simulink library "lib_converters"  (R2020b)
settings: Solver=VariableStepAuto  StartTime=0.0  StopTime=10.0  RelTol=1e-3
undefined symbols (not defined in the file): C_sc, DiscIntNeverNeededParam
libraries: powerlib x170, simulink x12, $bdroot x6, powerlib_meascontrol x3
(part 3 of 3)

== system lib_converters/Boost - FC/Discrete PI Controller3 ==
  note: Pierre Giroux, Gilbert Sybille
      | Power System Simulation Laboratory
      | IREQ, Hydro-Quebc
  note: Discrete PID Controller
  Error : Inport  SampleTime=Ts
  Discrete-Time Integrator : DiscreteIntegrator  InitialCondition=Init  SampleTime=Ts  LimitOutput=on  UpperSaturationLimit=UpperLimit  LowerSaturationLimit=LowerLimit  ICPrevOutput=DiscIntNeverNeededParam  ICPrevScaledInput=DiscIntNeverNeededParam
  Kp4 : Gain  Gain=Kp  SaturateOnIntegerOverflow=on  SampleTime=Ts  OutDataTypeStr=Inherit: Same as input  ParamDataTypeStr=Inherit: Same as input
  Kp5 : Gain  Gain=Ki  SaturateOnIntegerOverflow=on  SampleTime=Ts  OutDataTypeStr=Inherit: Same as input  ParamDataTypeStr=Inherit: Same as input
  Saturation2 : Saturate  UpperLimit=UpperLimit  LowerLimit=LowerLimit  SampleTime=Ts
  Sum6 : Sum  InputSameDT=on  SaturateOnIntegerOverflow=on  SampleTime=Ts  OutDataTypeStr=Inherit: Same as first input
  Zero-Order Hold : ZeroOrderHold  SampleTime=Ts
  Out : Outport  SampleTime=Ts  InitialOutput=0  VectorParamsAs1DForOutWhenUnconnected=off
  wires:
  Error/1 -> Kp4/1, Kp5/1
  Sum6/1 -> Saturation2/1
  Kp5/1 -> Discrete-Time Integrator/1
  Kp4/1 -> Zero-Order Hold/1
  Discrete-Time Integrator/1 -> Sum6/2
  Saturation2/1 -> Out/1
  Zero-Order Hold/1 -> Sum6/1

== system lib_converters/Boost - FC/Discrete PI Controller4 ==
  note: Discrete PID Controller
  note: Pierre Giroux, Gilbert Sybille
      | Power System Simulation Laboratory
      | IREQ, Hydro-Quebc
  Error : Inport  SampleTime=Ts
  Discrete-Time Integrator : DiscreteIntegrator  InitialCondition=Init  SampleTime=Ts  LimitOutput=on  UpperSaturationLimit=UpperLimit  LowerSaturationLimit=LowerLimit  ICPrevOutput=DiscIntNeverNeededParam  ICPrevScaledInput=DiscIntNeverNeededParam
  Kp4 : Gain  Gain=Kp  SaturateOnIntegerOverflow=on  SampleTime=Ts  OutDataTypeStr=Inherit: Same as input  ParamDataTypeStr=Inherit: Same as input
  Kp5 : Gain  Gain=Ki  SaturateOnIntegerOverflow=on  SampleTime=Ts  OutDataTypeStr=Inherit: Same as input  ParamDataTypeStr=Inherit: Same as input
  Saturation2 : Saturate  UpperLimit=UpperLimit  LowerLimit=LowerLimit  SampleTime=Ts
  Sum6 : Sum  InputSameDT=on  SaturateOnIntegerOverflow=on  SampleTime=Ts  OutDataTypeStr=Inherit: Same as first input
  Zero-Order Hold : ZeroOrderHold  SampleTime=Ts
  Out : Outport  SampleTime=Ts  InitialOutput=0  VectorParamsAs1DForOutWhenUnconnected=off
  wires:
  Zero-Order Hold/1 -> Sum6/1
  Saturation2/1 -> Out/1
  Discrete-Time Integrator/1 -> Sum6/2
  Kp4/1 -> Zero-Order Hold/1
  Kp5/1 -> Discrete-Time Integrator/1
  Sum6/1 -> Saturation2/1
  Error/1 -> Kp5/1, Kp4/1

== system lib_converters/Boost - PV/Control ==
  Vcom : Inport
  Icom : Inport  Port=2
  Vout : Inport  Port=3
  Iout : Inport  Port=4
  Vpv_in : Inport  Port=5
  IL : Inport  Port=6
  g : Inport  Port=7
  IR : Inport  Port=8
  Cascade-control : Subsystem  VariantControl=Cascade-control
  MPPT : Subsystem  VariantControl=MPPT
  Duty Cycle PV conv : Outport

== system lib_converters/Boost - PV - chsvar/Subsystem1 ==
  Vcom : Inport
  Icom : Inport  Port=2
  Vout : Inport  Port=3
  Iout : Inport  Port=4
  Vpv_in : Inport  Port=5
  IL : Inport  Port=6
  g : Inport  Port=7
  IR : Inport  Port=8
  Control : Inport  Port=9
  MATLAB Function : MATLAB Function  TreatAsAtomicUnit=on
  Saturation : Saturate  UpperLimit=1
  Subsystem : Subsystem
  Subsystem1 : Subsystem
  DutyCycle : Outport
  wires:
  Subsystem/1(Duty Cycle PV conv) -> MATLAB Function/2(mppt)
  Subsystem1/1(Duty Cycle PV conv) -> MATLAB Function/3(cascade)
  IR/1 -> [IR]
  g/1 -> [g]
  IL/1 -> [IL]
  Vpv_in/1 -> [Vpv_in]
  Iout/1 -> [Iout]
  Vout/1 -> [Vout]
  Icom/1 -> [Icom]
  Vcom/1 -> [Vcom]
  [Vcom] -> Subsystem/1(Vcom)
  [IR] -> Subsystem/8(IR)
  [Vout] -> Subsystem/3(Vout)
  [Icom] -> Subsystem/2(Icom)
  [g] -> Subsystem/7(g)
  [IL] -> Subsystem/6(IL)
  [Vpv_in] -> Subsystem/5(Vpv_in)
  [Iout] -> Subsystem/4(Iout)
  [Iout] -> Subsystem1/4(Iout)
  [Vpv_in] -> Subsystem1/5(Vpv_in)
  [IL] -> Subsystem1/6(IL)
  [g] -> Subsystem1/7(g)
  [Icom] -> Subsystem1/2(Icom)
  [Vout] -> Subsystem1/3(Vout)
  [IR] -> Subsystem1/8(IR)
  [Vcom] -> Subsystem1/1(Vcom)
  Saturation/1 -> DutyCycle/1
  MATLAB Function/1(d) -> Saturation/1
  Control/1 -> MATLAB Function/1(u1)

== system lib_converters/Boost FC avg-swh/Converter type ==
  g : Inport
  D : Inport  Port=2
  n : Inport  Port=3
  Avg : Subsystem  VariantControl=Choice
  Swh : Subsystem  VariantControl=Choice_1
  L+ : PMIOPort  Side=Left
  L- : PMIOPort  Port=2  Side=Left
  H+ : PMIOPort  Port=3  Side=Right
  H- : PMIOPort  Port=4  Side=Right
  VL : Outport
  IL : Outport  Port=2
  IR : Outport  Port=3
  VH : Outport  Port=4

== system lib_converters/Boost FC swh/Converter type ==
  g : Inport
  D : Inport  Port=2
  n : Inport  Port=3
  Avg : Subsystem  VariantControl=Choice
  Swh : Subsystem  VariantControl=Choice_1
  L+ : PMIOPort  Side=Left
  L- : PMIOPort  Port=2  Side=Left
  H+ : PMIOPort  Port=3  Side=Right
  H- : PMIOPort  Port=4  Side=Right
  VL : Outport
  IL : Outport  Port=2
  IR : Outport  Port=3
  VH : Outport  Port=4

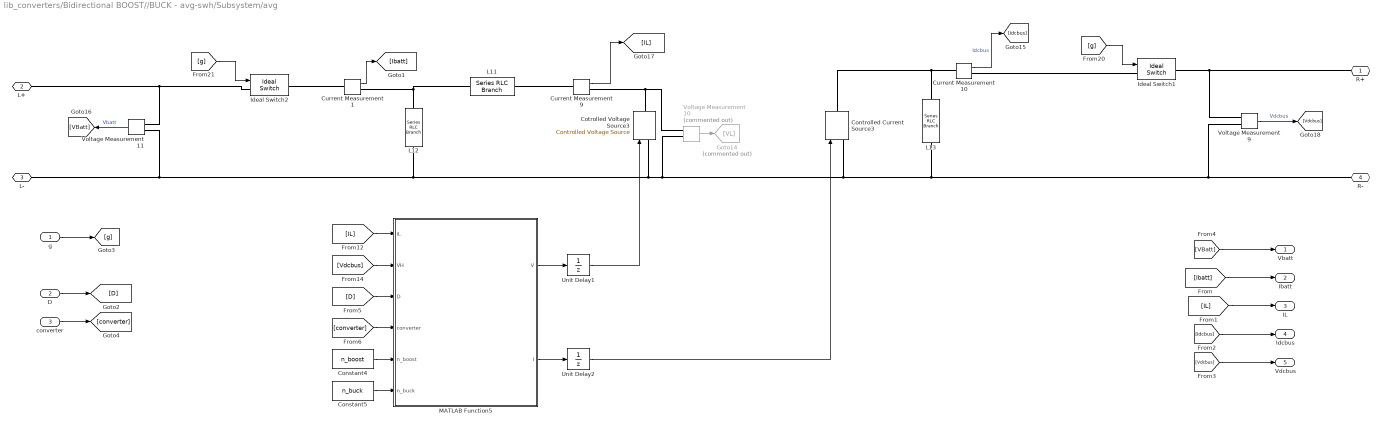
== system lib_converters/Bidirectional BOOST//BUCK - avg-swh/Subsystem/avg ==
  g : Inport
  D : Inport  Port=2
  converter : Inport  Port=3
  Constant4 : Constant  Value=n_boost
  Constant5 : Constant  Value=n_buck
  Controlled Current Source3 : powerlib/Electrical Sources/Controlled Current Source  Initialize=on  Source_Type=DC  Amplitude=0  Phase=0  Frequency=0  Measurements=None
  Cotrolled Voltage Source3 : powerlib/Electrical Sources/Controlled Voltage Source  Initialize=on  Source_Type=DC  Amplitude=0  Phase=0  Frequency=0  Measurements=None
  Current Measurement1 : powerlib/Measurements/Current Measurement  PhasorSimulation=off  OutputType=Complex  PSBequivalent=0
  Current Measurement10 : powerlib/Measurements/Current Measurement  PhasorSimulation=off  OutputType=Complex  PSBequivalent=0
  Current Measurement9 : powerlib/Measurements/Current Measurement  PhasorSimulation=off  OutputType=Complex  PSBequivalent=0
  Goto14 : Goto  Commented=on  GotoTag=VL
  Ideal Switch1 : powerlib/Power Electronics/Ideal Switch  Ron=0.001  Lon=0  IC=0  Rs=1e5  Cs=inf  Measurements=off
  Ideal Switch2 : powerlib/Power Electronics/Ideal Switch  Ron=0.001  Lon=0  IC=0  Rs=1e5  Cs=inf  Measurements=off
  L11 : powerlib/Elements/Series RLC Branch  LConnTagsString=__new0  RConnTagsString=__new0  BranchType=L  Resistance=0.3  Inductance=L  SetiL0=off  InitialCurrent=100  Capacitance=100e-6  Setx0=off  InitialVoltage=0  Measurements=None
  L12 : powerlib/Elements/Series RLC Branch  LConnTagsString=__new0  RConnTagsString=__new0  BranchType=RC  Resistance=0.01  Inductance=100e-6  SetiL0=off  InitialCurrent=100  Capacitance=Co  Setx0=off  InitialVoltage=0  Measurements=None
  L13 : powerlib/Elements/Series RLC Branch  LConnTagsString=__new0  RConnTagsString=__new0  BranchType=RC  Resistance=0.01  Inductance=100e-6  SetiL0=off  InitialCurrent=100  Capacitance=Co  Setx0=off  InitialVoltage=0  Measurements=None
  MATLAB Function5 : MATLAB Function  TreatAsAtomicUnit=on
  Unit Delay1 : UnitDelay  SampleTime=Ts  HasFrameUpgradeWarning=on
  Unit Delay2 : UnitDelay  SampleTime=Ts  HasFrameUpgradeWarning=on
  Voltage Measurement10 : powerlib/Measurements/Voltage Measurement  Commented=on  PhasorSimulation=off  OutputType=Complex  PSBequivalent=0
  Voltage Measurement11 : powerlib/Measurements/Voltage Measurement  PhasorSimulation=off  OutputType=Complex  PSBequivalent=0
  Voltage Measurement9 : powerlib/Measurements/Voltage Measurement  PhasorSimulation=off  OutputType=Complex  PSBequivalent=0
  R+ : PMIOPort  Side=Right
  L+ : PMIOPort  Port=2  Side=Left
  L- : PMIOPort  Port=3  Side=Left
  R- : PMIOPort  Port=4  Side=Right
  Vbatt : Outport
  Ibatt : Outport  Port=2
  IL : Outport  Port=3
  Idcbus : Outport  Port=4
  Vdcbus : Outport  Port=5
  wires:
  [g] -> Ideal Switch1/1
  MATLAB Function5/2(I) -> Unit Delay2/1
  Current Measurement1/1 -> [Ibatt]
  [D] -> MATLAB Function5/3(D)
  Voltage Measurement11/1 -> [VBatt]  "Vbatt"
  Unit Delay2/1 -> Controlled Current Source3/1
  Voltage Measurement9/1 -> [Vdcbus]  "Vdcbus"
  [converter] -> MATLAB Function5/4(converter)
  [Vdcbus] -> MATLAB Function5/2(VH)
  Constant4/1 -> MATLAB Function5/5(n_boost)
  [g] -> Ideal Switch2/1
  [IL] -> MATLAB Function5/1(iL)
  MATLAB Function5/1(V) -> Unit Delay1/1
  Unit Delay1/1 -> Cotrolled Voltage Source3/1
  Current Measurement9/1 -> [IL]
  Voltage Measurement10/1 -> Goto14/1
  Constant5/1 -> MATLAB Function5/6(n_buck)
  Current Measurement10/1 -> [Idcbus]  "Idcbus"
  g/1 -> [g]
  converter/1 -> [converter]
  D/1 -> [D]
  [VBatt] -> Vbatt/1
  [Ibatt] -> Ibatt/1
  [IL] -> IL/1
  [Idcbus] -> Idcbus/1
  [Vdcbus] -> Vdcbus/1
  connections:
  Voltage Measurement9/LConn2 -- R-/RConn1 -- L13/RConn1 -- Controlled Current Source3/LConn1 -- Voltage Measurement10/LConn2 -- Cotrolled Voltage Source3/LConn1 -- L-/RConn1 -- Voltage Measurement11/LConn2 -- L12/RConn1
  Controlled Current Source3/RConn1 -- Current Measurement10/LConn1 -- L13/LConn1
  Current Measurement1/RConn1 -- L12/LConn1 -- L11/RConn1
  Voltage Measurement10/LConn1 -- Cotrolled Voltage Source3/RConn1 -- Current Measurement9/RConn1
  R+/RConn1 -- Ideal Switch1/RConn1 -- Voltage Measurement9/LConn1
  Ideal Switch2/LConn1 -- L+/RConn1 -- Voltage Measurement11/LConn1
  Ideal Switch1/LConn1 -- Current Measurement10/RConn1
  Current Measurement9/LConn1 -- L11/LConn1
  Ideal Switch2/RConn1 -- Current Measurement1/LConn1

== system lib_converters/Bidirectional BOOST//BUCK - avg-swh/Subsystem/swh ==
  g : Inport
  D : Inport  Port=2
  converter : Inport  Port=3
  Current Measurement1 : powerlib/Measurements/Current Measurement  PhasorSimulation=off  OutputType=Complex  PSBequivalent=0
  Current Measurement10 : powerlib/Measurements/Current Measurement  PhasorSimulation=off  OutputType=Complex  PSBequivalent=0
  Current Measurement9 : powerlib/Measurements/Current Measurement  PhasorSimulation=off  OutputType=Complex  PSBequivalent=0
  Ideal Switch1 : powerlib/Power Electronics/Ideal Switch  Ron=0.001  Lon=0  IC=0  Rs=1e5  Cs=inf  Measurements=off
  Ideal Switch2 : powerlib/Power Electronics/Ideal Switch  Ron=0.001  Lon=0  IC=0  Rs=1e5  Cs=inf  Measurements=off
  L11 : powerlib/Elements/Series RLC Branch  LConnTagsString=__new0  RConnTagsString=__new0  BranchType=L  Resistance=0.3  Inductance=L  SetiL0=off  InitialCurrent=100  Capacitance=100e-6  Setx0=off  InitialVoltage=0  Measurements=None
  L12 : powerlib/Elements/Series RLC Branch  LConnTagsString=__new0  RConnTagsString=__new0  BranchType=RC  Resistance=0.01  Inductance=100e-6  SetiL0=off  InitialCurrent=100  Capacitance=Co  Setx0=off  InitialVoltage=0  Measurements=None
  L13 : powerlib/Elements/Series RLC Branch  LConnTagsString=__new0  RConnTagsString=__new0  BranchType=RC  Resistance=0.01  Inductance=100e-6  SetiL0=off  InitialCurrent=100  Capacitance=Co  Setx0=off  InitialVoltage=0  Measurements=None
  Mosfet : powerlib/Power Electronics/Mosfet  Ron=0.1  Lon=0  Rd=0.01  Vfd=0  IC=0  Rs=1e5  Cs=inf  Measurements=on
  Mosfet1 : powerlib/Power Electronics/Mosfet  Ron=0.1  Lon=0  Rd=0.01  Vfd=0  IC=0  Rs=1e5  Cs=inf  Measurements=on
  NOT : Logic  Operator=NOT  IconShape=distinctive  AllPortsSameDT=off  OutDataTypeStr=boolean
  PWM Generator (DC-DC) : powerlib_meascontrol/Pulse & Signal Generators/PWM Generator (DC-DC)  Fsw=100000  Ts=Ts
  Product : Product
  Product1 : Product
  Voltage Measurement11 : powerlib/Measurements/Voltage Measurement  PhasorSimulation=off  OutputType=Complex  PSBequivalent=0
  Voltage Measurement9 : powerlib/Measurements/Voltage Measurement  PhasorSimulation=off  OutputType=Complex  PSBequivalent=0
  R+ : PMIOPort  Side=Right
  L+ : PMIOPort  Port=2  Side=Left
  L- : PMIOPort  Port=3  Side=Left
  R- : PMIOPort  Port=4  Side=Right
  Vbatt : Outport
  Ibatt : Outport  Port=2
  IL : Outport  Port=3
  Idcbus : Outport  Port=4
  Vdcbus : Outport  Port=5
  wires:
  Current Measurement9/1 -> [IL]
  [g] -> Ideal Switch2/1
  Voltage Measurement11/1 -> [VBatt]  "Vbatt"
  [g] -> Ideal Switch1/1
  Voltage Measurement9/1 -> [Vdcbus]  "Vdcbus"
  Current Measurement1/1 -> [Ibatt]
  D/1 -> [D]
  Current Measurement10/1 -> [Idcbus]  "Idcbus"
  g/1 -> [g]
  [Idcbus] -> Idcbus/1
  [Ibatt] -> Ibatt/1
  [Vdcbus] -> Vdcbus/1
  [IL] -> IL/1
  [VBatt] -> Vbatt/1
  converter/1 -> [converter]
  [D] -> PWM Generator (DC-DC)/1
  PWM Generator (DC-DC)/1 -> Product1/1, Product/1
  [converter] -> NOT/1, Product/2
  NOT/1 -> Product1/2
  Product1/1 -> Mosfet1/1
  Product/1 -> Mosfet/1
  connections:
  L12/RConn1 -- Mosfet1/RConn1 -- L13/RConn1 -- R-/RConn1 -- Voltage Measurement9/LConn2 -- L-/RConn1 -- Voltage Measurement11/LConn2
  R+/RConn1 -- Ideal Switch1/RConn1 -- Voltage Measurement9/LConn1
  Current Measurement1/RConn1 -- L12/LConn1 -- L11/RConn1
  Ideal Switch2/LConn1 -- L+/RConn1 -- Voltage Measurement11/LConn1
  L13/LConn1 -- Current Measurement10/LConn1 -- Mosfet/LConn1
  Current Measurement9/LConn1 -- L11/LConn1
  Ideal Switch1/LConn1 -- Current Measurement10/RConn1
  Ideal Switch2/RConn1 -- Current Measurement1/LConn1
  Mosfet1/LConn1 -- Mosfet/RConn1 -- Current Measurement9/RConn1

== system lib_converters/Boost - PV/Control/Cascade-control ==
  note: Current Regulator
  note: Voltage Regulator
  Vcom : Inport
  Icom : Inport  Port=2
  Vout : Inport  Port=3
  Iout : Inport  Port=4
  Vpv_in : Inport  Port=5
  IL : Inport  Port=6
  g : Inport  Port=7
  IR : Inport  Port=8
  Constant : Constant
  Constant1 : Constant  Value=0
  Constant8 : Constant  Value=n
  Discrete PI Controller3 : Subsystem  DialogController=POWERSYS.PowerSysDialog  mask(Discrete PI Controller){Kp=Kpv, Ki=Kiv, Par_Limits=[0.5 -0.5], Init=0, Ts=Ts}
      mask prompts: Kp "Proportional gain (Kp):"; Ki "Integral gain (Ki):"; Par_Limits "Output limits: [ Upper   Lower ]"; Init "Output initial value:"; Ts "Sample time:"
      mask help: This block implements a discrete PI controller.
      mask init:
      | UpperLimit=Par_Limits(1);
      | LowerLimit=Par_Limits(2);
      | power_initmask();
      mask Help: This block is part of a subset of blocks in the Extras library that does not have documentation associated with it, other than the block mask description.
      mask Display: disp('PI');
  Discrete PI Controller4 : Subsystem  DialogController=POWERSYS.PowerSysDialog  mask(Discrete PI Controller){Kp=Kpi, Ki=Kii, Par_Limits=[50 -50], Init=0, Ts=Ts}
      mask prompts: Kp "Proportional gain (Kp):"; Ki "Integral gain (Ki):"; Par_Limits "Output limits: [ Upper   Lower ]"; Init "Output initial value:"; Ts "Sample time:"
      mask help: This block implements a discrete PI controller.
      mask init:
      | UpperLimit=Par_Limits(1);
      | LowerLimit=Par_Limits(2);
      | power_initmask();
      mask Help: This block is part of a subset of blocks in the Extras library that does not have documentation associated with it, other than the block mask description.
      mask Display: disp('PI');
  Divide : Product  Inputs=*/  SampleTime=Ts
  Divide1 : Product  Inputs=*/  SampleTime=Ts
  Product : Product  RndMeth=Zero
  Product1 : Product  RndMeth=Zero
  Product2 : Product  RndMeth=Zero
  Saturation : Saturate  UpperLimit=inf  LowerLimit=0.01  SampleTime=Ts
  Saturation Dynamic : simulink/Discontinuities/Saturation Dynamic  OutMin=[]  OutMax=[]  OutDataTypeStr=Inherit: Same as second input  OutDataType=fixdt(1, 16)  OutScaling=2^-10  DoSatur=off
  Saturation1 : Saturate  UpperLimit=1  LowerLimit=0  SampleTime=Ts
  Saturation2 : Saturate  UpperLimit=inf  LowerLimit=0.01  SampleTime=Ts
  Sum : Sum  Inputs=|+-
  Sum1 : Sum  Inputs=|-+
  Sum2 : Sum  Inputs=|-+
  Sum3 : Sum  Inputs=|+-
  Sum4 : Sum  Inputs=|++
  Duty Cycle PV conv : Outport
  wires:
  Vout/1 -> [VH]
  Iout/1 -> ?
  IL/1 -> [IL]
  Vpv_in/1 -> [VL]
  Saturation1/1 -> Duty Cycle PV conv/1  "Duty Cycle PV conv"
  Vcom/1 -> Sum3/1
  Constant8/1 -> Product2/2
  Divide/1 -> Sum2/1
  Icom/1 -> Product1/1
  Discrete PI Controller3/1(Out) -> Sum4/1
  Product2/1 -> Saturation2/1
  Sum4/1 -> Product/1
  [IL] -> Sum/2
  Saturation/1 -> Divide/2
  Saturation2/1 -> Divide1/2
  [VH] -> Saturation/1
  Saturation Dynamic/1 -> [ILref]
  [IR] -> Sum4/2
  Divide1/1 -> Product/2
  [VL] -> Sum1/2
  [ILref] -> Sum/1
  [VH] -> Divide1/1
  [VH] -> Sum3/2
  Product/1 -> Saturation Dynamic/2
  Sum/1 -> Discrete PI Controller4/1(Error)
  Discrete PI Controller4/1(Out) -> Sum1/1
  Constant1/1 -> Saturation Dynamic/3
  Sum2/1 -> Saturation1/1
  Constant/1 -> Sum2/2
  [g] -> Product1/2
  Sum3/1 -> Discrete PI Controller3/1(Error)
  Sum1/1 -> Divide/1
  Product1/1 -> Saturation Dynamic/1
  [VL] -> Product2/1
  IR/1 -> [IR]
  g/1 -> [g]

== system lib_converters/Boost - PV/Control/MPPT ==
  Vcom : Inport
  Icom : Inport  Port=2
  Vout : Inport  Port=3
  Iout : Inport  Port=4
  Vpv_in : Inport  Port=5
  IL : Inport  Port=6
  g : Inport  Port=7
  IR : Inport  Port=8
  MPPT : MATLAB Function  TreatAsAtomicUnit=on
  Saturation1 : Saturate  UpperLimit=1  LowerLimit=0  SampleTime=Ts
  Unit Delay1 : UnitDelay  SampleTime=Ts*10  HasFrameUpgradeWarning=on
  Duty Cycle PV conv : Outport
  wires:
  Icom/1 -> MPPT/2(Icom)
  Vpv_in/1 -> MPPT/5(Vpv_in)
  Vout/1 -> MPPT/3(Vout)
  Saturation1/1 -> Duty Cycle PV conv/1  "Duty Cycle PV conv"
  Vcom/1 -> MPPT/1(Vcom)
  Unit Delay1/1 -> Saturation1/1
  MPPT/1(D) -> Unit Delay1/1
  Iout/1 -> MPPT/4(Iout)
  IL/1 -> MPPT/6(I_L)

== system lib_converters/Boost - PV - chsvar/Subsystem1/Subsystem ==
  Vcom : Inport
  Icom : Inport  Port=2
  Vout : Inport  Port=3
  Iout : Inport  Port=4
  Vpv_in : Inport  Port=5
  IL : Inport  Port=6
  g : Inport  Port=7
  IR : Inport  Port=8
  MPPT : MATLAB Function  TreatAsAtomicUnit=on
  Saturation1 : Saturate  UpperLimit=1  LowerLimit=0  SampleTime=Ts
  Terminator : Terminator
  Terminator1 : Terminator
  Unit Delay2 : UnitDelay  SampleTime=Ts*10  HasFrameUpgradeWarning=on
  Duty Cycle PV conv : Outport
  wires:
  IL/1 -> MPPT/6(I_L)
  Unit Delay2/1 -> Saturation1/1
  Vout/1 -> MPPT/3(Vout)
  Vcom/1 -> MPPT/1(Vcom)
  Iout/1 -> MPPT/4(Iout)
  Vpv_in/1 -> MPPT/5(Vpv_in)
  Saturation1/1 -> Duty Cycle PV conv/1  "Duty Cycle PV conv"
  MPPT/1(D) -> Unit Delay2/1
  Icom/1 -> MPPT/2(Icom)
  g/1 -> Terminator/1
  IR/1 -> Terminator1/1

== system lib_converters/Boost - PV - chsvar/Subsystem1/Subsystem1 ==
  note: Current Regulator
  note: Voltage Regulator
  Vcom : Inport
  Icom : Inport  Port=2
  Vout : Inport  Port=3
  Iout : Inport  Port=4
  Vpv_in : Inport  Port=5
  IL : Inport  Port=6
  g : Inport  Port=7
  IR : Inport  Port=8
  Constant : Constant
  Constant1 : Constant  Value=0
  Constant8 : Constant  Value=n
  Discrete PI Controller3 : Subsystem  DialogController=POWERSYS.PowerSysDialog  mask(Discrete PI Controller){Kp=Kpv, Ki=Kiv, Par_Limits=[0.5 -0.5], Init=0, Ts=Ts}
      mask prompts: Kp "Proportional gain (Kp):"; Ki "Integral gain (Ki):"; Par_Limits "Output limits: [ Upper   Lower ]"; Init "Output initial value:"; Ts "Sample time:"
      mask help: This block implements a discrete PI controller.
      mask init:
      | UpperLimit=Par_Limits(1);
      | LowerLimit=Par_Limits(2);
      | power_initmask();
      mask Help: This block is part of a subset of blocks in the Extras library that does not have documentation associated with it, other than the block mask description.
      mask Display: disp('PI');
  Discrete PI Controller4 : Subsystem  DialogController=POWERSYS.PowerSysDialog  mask(Discrete PI Controller){Kp=Kpi, Ki=Kii, Par_Limits=[50 -50], Init=0, Ts=Ts}
      mask prompts: Kp "Proportional gain (Kp):"; Ki "Integral gain (Ki):"; Par_Limits "Output limits: [ Upper   Lower ]"; Init "Output initial value:"; Ts "Sample time:"
      mask help: This block implements a discrete PI controller.
      mask init:
      | UpperLimit=Par_Limits(1);
      | LowerLimit=Par_Limits(2);
      | power_initmask();
      mask Help: This block is part of a subset of blocks in the Extras library that does not have documentation associated with it, other than the block mask description.
      mask Display: disp('PI');
  Divide : Product  Inputs=*/  SampleTime=Ts
  Divide1 : Product  Inputs=*/  SampleTime=Ts
  Product : Product  RndMeth=Zero
  Product1 : Product  RndMeth=Zero
  Product2 : Product  RndMeth=Zero
  Saturation : Saturate  UpperLimit=inf  LowerLimit=0.01  SampleTime=Ts
  Saturation Dynamic : simulink/Discontinuities/Saturation Dynamic  OutMin=[]  OutMax=[]  OutDataTypeStr=Inherit: Same as second input  OutDataType=fixdt(1, 16)  OutScaling=2^-10  DoSatur=off
  Saturation1 : Saturate  UpperLimit=1  LowerLimit=0  SampleTime=Ts
  Saturation2 : Saturate  UpperLimit=inf  LowerLimit=0.01  SampleTime=Ts
  Sum : Sum  Inputs=|+-
  Sum1 : Sum  Inputs=|-+
  Sum2 : Sum  Inputs=|-+
  Sum3 : Sum  Inputs=|+-
  Sum4 : Sum  Inputs=|++
  Terminator : Terminator
  Duty Cycle PV conv : Outport
  wires:
  Iout/1 -> Terminator/1
  Sum3/1 -> Discrete PI Controller3/1(Error)
  Discrete PI Controller4/1(Out) -> Sum1/1
  Constant1/1 -> Saturation Dynamic/3
  IR/1 -> [IR]
  [VL] -> Product2/1
  Divide1/1 -> Product/2
  Product1/1 -> Saturation Dynamic/1
  Product2/1 -> Saturation2/1
  [IR] -> Sum4/2
  Sum2/1 -> Saturation1/1
  [VH] -> Saturation/1
  Constant/1 -> Sum2/2
  [g] -> Product1/2
  Saturation2/1 -> Divide1/2
  [ILref] -> Sum/1
  [IL] -> Sum/2
  [VH] -> Divide1/1
  [VL] -> Sum1/2
  Saturation/1 -> Divide/2
  Sum4/1 -> Product/1
  Constant8/1 -> Product2/2
  Product/1 -> Saturation Dynamic/2
  g/1 -> [g]
  IL/1 -> [IL]
  Icom/1 -> Product1/1
  Saturation Dynamic/1 -> [ILref]
  Vcom/1 -> Sum3/1
  Saturation1/1 -> Duty Cycle PV conv/1  "Duty Cycle PV conv"
  Divide/1 -> Sum2/1
  [VH] -> Sum3/2
  Vpv_in/1 -> [VL]
  Vout/1 -> [VH]
  Sum1/1 -> Divide/1
  Discrete PI Controller3/1(Out) -> Sum4/1
  Sum/1 -> Discrete PI Controller4/1(Error)

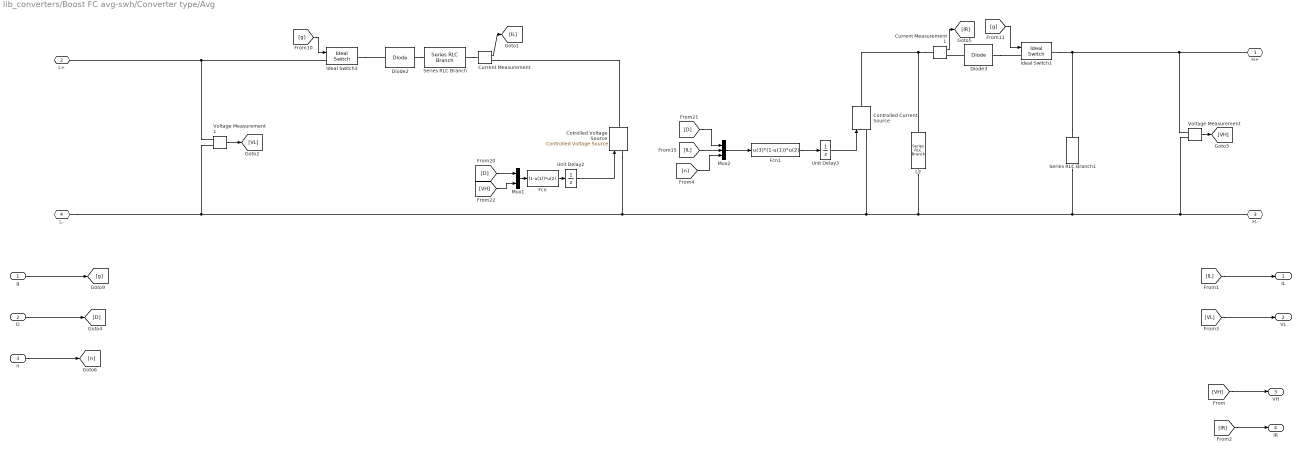
== system lib_converters/Boost FC avg-swh/Converter type/Avg ==
  g : Inport
  D : Inport  Port=2
  n : Inport  Port=3
  Controlled Current Source : powerlib/Electrical Sources/Controlled Current Source  Initialize=off  Source_Type=DC  Amplitude=0  Phase=0  Frequency=0  Measurements=None
  Cotrolled Voltage Source : powerlib/Electrical Sources/Controlled Voltage Source  Initialize=off  Source_Type=DC  Amplitude=0  Phase=0  Frequency=0  Measurements=None
  Current Measurement : powerlib/Measurements/Current Measurement  PhasorSimulation=off  OutputType=Complex  PSBequivalent=0
  Current Measurement1 : powerlib/Measurements/Current Measurement  PhasorSimulation=off  OutputType=Complex  PSBequivalent=0
  Diode2 : powerlib/Power Electronics/Diode  Ron=0.001  Lon=0  Vf=0  IC=0  UseSnubber=off  Rs=1e6  Cs=250e-9  Measurements=off
  Diode3 : powerlib/Power Electronics/Diode  Ron=0.001  Lon=0  Vf=0  IC=0  UseSnubber=off  Rs=1e6  Cs=250e-9  Measurements=off
  Fcn : Fcn  Expr=(1-u(1))*u(2)
  Fcn1 : Fcn  Expr=u(3)*(1-u(1))*u(2)
  Ideal Switch1 : powerlib/Power Electronics/Ideal Switch  Ron=0.001  Lon=0  IC=0  Rs=1e5  Cs=inf  Measurements=off
  Ideal Switch3 : powerlib/Power Electronics/Ideal Switch  Ron=0.001  Lon=0  IC=0  Rs=1e5  Cs=inf  Measurements=off
  L2 : powerlib/Elements/Series RLC Branch  LConnTagsString=__new0  RConnTagsString=__new0  BranchType=C  Resistance=0.01  Inductance=100e-6  SetiL0=off  InitialCurrent=100  Capacitance=Co  Setx0=off  InitialVoltage=100  Measurements=None
  Mux1 : Mux  Inputs=2
  Mux2 : Mux  Inputs=3
  Series RLC Branch : powerlib/Elements/Series RLC Branch  LConnTagsString=__new0  RConnTagsString=__new0  BranchType=L  Resistance=1  Inductance=L  SetiL0=off  InitialCurrent=1  Capacitance=1e-6  Setx0=off  InitialVoltage=0  Measurements=None
  Series RLC Branch1 : powerlib/Elements/Series RLC Branch  LConnTagsString=__new0  RConnTagsString=__new0  BranchType=R  Resistance=5e3  Inductance=1e-3  SetiL0=off  InitialCurrent=0  Capacitance=15  Setx0=on  InitialVoltage=270  Measurements=None
  Unit Delay2 : UnitDelay  SampleTime=Ts  HasFrameUpgradeWarning=on
  Unit Delay3 : UnitDelay  SampleTime=Ts  HasFrameUpgradeWarning=on
  Voltage Measurement : powerlib/Measurements/Voltage Measurement  PhasorSimulation=off  OutputType=Complex  PSBequivalent=0
  Voltage Measurement1 : powerlib/Measurements/Voltage Measurement  PhasorSimulation=off  OutputType=Complex  PSBequivalent=0
  H+ : PMIOPort  Side=Right
  L+ : PMIOPort  Port=2  Side=Left
  H- : PMIOPort  Port=3  Side=Right
  L- : PMIOPort  Port=4  Side=Left
  IL : Outport
  VL : Outport  Port=2
  VH : Outport  Port=3
  IR : Outport  Port=4
  wires:
  [D] -> Mux1/1
  Voltage Measurement1/1 -> [VL]
  Unit Delay3/1 -> Controlled Current Source/1
  [n] -> Mux2/3
  Fcn1/1 -> Unit Delay3/1
  [IL] -> Mux2/2
  Current Measurement1/1 -> [IR]
  Mux1/1 -> Fcn/1
  Mux2/1 -> Fcn1/1
  g/1 -> [g]
  Unit Delay2/1 -> Cotrolled Voltage Source/1
  [g] -> Ideal Switch3/1
  Current Measurement/1 -> [IL]
  [VH] -> Mux1/2
  Voltage Measurement/1 -> [VH]
  [D] -> Mux2/1
  Fcn/1 -> Unit Delay2/1
  [g] -> Ideal Switch1/1
  [IR] -> IR/1
  [VH] -> VH/1
  [VL] -> VL/1
  [IL] -> IL/1
  n/1 -> [n]
  D/1 -> [D]
  connections:
  Series RLC Branch1/LConn1 -- Ideal Switch1/RConn1 -- H+/RConn1 -- Voltage Measurement/LConn1
  L+/RConn1 -- Ideal Switch3/LConn1 -- Voltage Measurement1/LConn1
  Current Measurement1/LConn1 -- L2/LConn1 -- Controlled Current Source/RConn1
  Series RLC Branch1/RConn1 -- Controlled Current Source/LConn1 -- Cotrolled Voltage Source/LConn1 -- Voltage Measurement1/LConn2 -- L-/RConn1 -- L2/RConn1 -- H-/RConn1 -- Voltage Measurement/LConn2
  Current Measurement/RConn1 -- Cotrolled Voltage Source/RConn1
  Ideal Switch3/RConn1 -- Diode2/LConn1
  Series RLC Branch/RConn1 -- Current Measurement/LConn1
  Diode3/RConn1 -- Ideal Switch1/LConn1
  Diode3/LConn1 -- Current Measurement1/RConn1
  Diode2/RConn1 -- Series RLC Branch/LConn1

== system lib_converters/Boost FC avg-swh/Converter type/Swh ==
  g : Inport
  D : Inport  Port=2
  n : Inport  Port=3
  Current Measurement : powerlib/Measurements/Current Measurement  PhasorSimulation=off  OutputType=Complex  PSBequivalent=0
  Current Measurement1 : powerlib/Measurements/Current Measurement  PhasorSimulation=off  OutputType=Complex  PSBequivalent=0
  Diode1 : powerlib/Power Electronics/Diode  Ron=0.001  Lon=0  Vf=0  IC=0  UseSnubber=off  Rs=1e6  Cs=250e-9  Measurements=off
  Diode2 : powerlib/Power Electronics/Diode  Ron=0.001  Lon=0  Vf=0  IC=0  UseSnubber=off  Rs=1e6  Cs=250e-9  Measurements=off
  Diode3 : powerlib/Power Electronics/Diode  Ron=0.001  Lon=0  Vf=0  IC=0  UseSnubber=off  Rs=1e6  Cs=250e-9  Measurements=off
  Ideal Switch1 : powerlib/Power Electronics/Ideal Switch  Ron=0.001  Lon=0  IC=0  Rs=1e5  Cs=inf  Measurements=off
  Ideal Switch3 : powerlib/Power Electronics/Ideal Switch  Ron=0.001  Lon=0  IC=0  Rs=1e5  Cs=inf  Measurements=off
  L2 : powerlib/Elements/Series RLC Branch  LConnTagsString=__new0  RConnTagsString=__new0  BranchType=C  Resistance=0.01  Inductance=100e-6  SetiL0=off  InitialCurrent=100  Capacitance=Co  Setx0=off  InitialVoltage=100  Measurements=None
  Mosfet : powerlib/Power Electronics/Mosfet  Ron=0.1  Lon=0  Rd=0.01  Vfd=0  IC=0  Rs=1e5  Cs=inf  Measurements=on
  PWM Generator (DC-DC) : powerlib_meascontrol/Pulse & Signal Generators/PWM Generator (DC-DC)  Fsw=10000  Ts=Ts
  Series RLC Branch : powerlib/Elements/Series RLC Branch  LConnTagsString=__new0  RConnTagsString=__new0  BranchType=L  Resistance=1  Inductance=L  SetiL0=off  InitialCurrent=1  Capacitance=1e-6  Setx0=off  InitialVoltage=0  Measurements=None
  Series RLC Branch1 : powerlib/Elements/Series RLC Branch  LConnTagsString=__new0  RConnTagsString=__new0  BranchType=R  Resistance=5e3  Inductance=1e-3  SetiL0=off  InitialCurrent=0  Capacitance=15  Setx0=on  InitialVoltage=270  Measurements=None
  Voltage Measurement : powerlib/Measurements/Voltage Measurement  PhasorSimulation=off  OutputType=Complex  PSBequivalent=0
  Voltage Measurement1 : powerlib/Measurements/Voltage Measurement  PhasorSimulation=off  OutputType=Complex  PSBequivalent=0
  H+ : PMIOPort  Side=Right
  L+ : PMIOPort  Port=2  Side=Left
  H- : PMIOPort  Port=3  Side=Right
  L- : PMIOPort  Port=4  Side=Left
  IL : Outport
  VL : Outport  Port=2
  VH : Outport  Port=3
  IR : Outport  Port=4
  wires:
  [IR] -> IR/1
  [VH] -> VH/1
  [VL] -> VL/1
  [g] -> Ideal Switch1/1
  Current Measurement1/1 -> [IR]
  g/1 -> [g]
  Voltage Measurement/1 -> [VH]
  [IL] -> IL/1
  Current Measurement/1 -> [IL]
  [g] -> Ideal Switch3/1
  n/1 -> [n]
  Voltage Measurement1/1 -> [VL]
  D/1 -> [D]
  [D] -> PWM Generator (DC-DC)/1
  PWM Generator (DC-DC)/1 -> Mosfet/1
  connections:
  Voltage Measurement/LConn2 -- H-/RConn1 -- Series RLC Branch1/RConn1 -- Voltage Measurement1/LConn2 -- L-/RConn1 -- Mosfet/RConn1 -- L2/RConn1
  Voltage Measurement1/LConn1 -- L+/RConn1 -- Ideal Switch3/LConn1
  Voltage Measurement/LConn1 -- H+/RConn1 -- Ideal Switch1/RConn1 -- Series RLC Branch1/LConn1
  Diode2/RConn1 -- Series RLC Branch/LConn1
  Ideal Switch3/RConn1 -- Diode2/LConn1
  Series RLC Branch/RConn1 -- Current Measurement/LConn1
  Mosfet/LConn1 -- Current Measurement/RConn1 -- Diode1/LConn1
  Current Measurement1/LConn1 -- L2/LConn1 -- Diode1/RConn1
  Diode3/RConn1 -- Ideal Switch1/LConn1
  Diode3/LConn1 -- Current Measurement1/RConn1

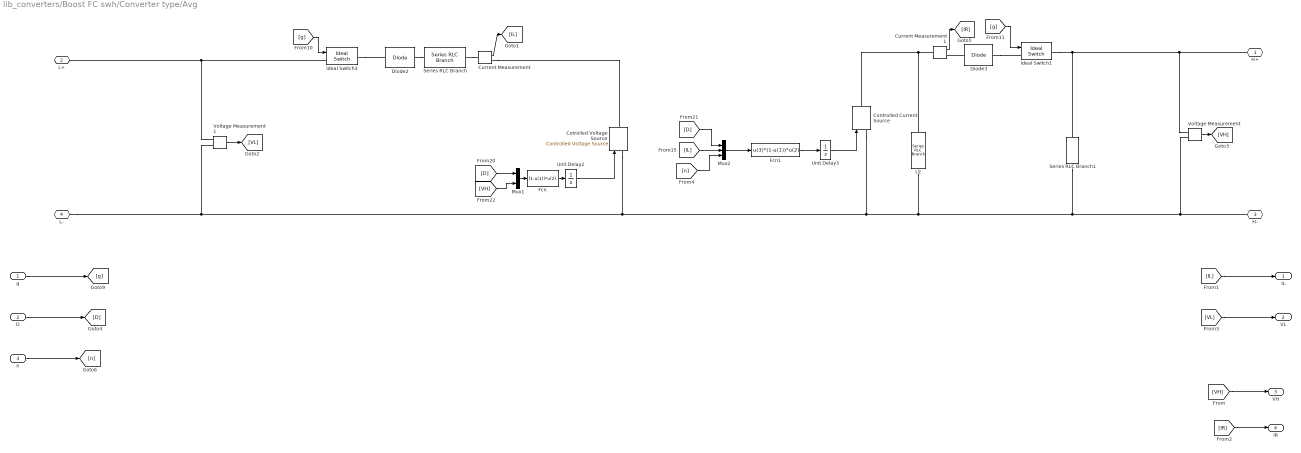
== system lib_converters/Boost FC swh/Converter type/Avg ==
  g : Inport
  D : Inport  Port=2
  n : Inport  Port=3
  Controlled Current Source : powerlib/Electrical Sources/Controlled Current Source  Initialize=off  Source_Type=DC  Amplitude=0  Phase=0  Frequency=0  Measurements=None
  Cotrolled Voltage Source : powerlib/Electrical Sources/Controlled Voltage Source  Initialize=off  Source_Type=DC  Amplitude=0  Phase=0  Frequency=0  Measurements=None
  Current Measurement : powerlib/Measurements/Current Measurement  PhasorSimulation=off  OutputType=Complex  PSBequivalent=0
  Current Measurement1 : powerlib/Measurements/Current Measurement  PhasorSimulation=off  OutputType=Complex  PSBequivalent=0
  Diode2 : powerlib/Power Electronics/Diode  Ron=0.001  Lon=0  Vf=0  IC=0  UseSnubber=off  Rs=1e6  Cs=250e-9  Measurements=off
  Diode3 : powerlib/Power Electronics/Diode  Ron=0.001  Lon=0  Vf=0  IC=0  UseSnubber=off  Rs=1e6  Cs=250e-9  Measurements=off
  Fcn : Fcn  Expr=(1-u(1))*u(2)
  Fcn1 : Fcn  Expr=u(3)*(1-u(1))*u(2)
  Ideal Switch1 : powerlib/Power Electronics/Ideal Switch  Ron=0.001  Lon=0  IC=0  Rs=1e5  Cs=inf  Measurements=off
  Ideal Switch3 : powerlib/Power Electronics/Ideal Switch  Ron=0.001  Lon=0  IC=0  Rs=1e5  Cs=inf  Measurements=off
  L2 : powerlib/Elements/Series RLC Branch  LConnTagsString=__new0  RConnTagsString=__new0  BranchType=C  Resistance=0.01  Inductance=100e-6  SetiL0=off  InitialCurrent=100  Capacitance=Co  Setx0=off  InitialVoltage=100  Measurements=None
  Mux1 : Mux  Inputs=2
  Mux2 : Mux  Inputs=3
  Series RLC Branch : powerlib/Elements/Series RLC Branch  LConnTagsString=__new0  RConnTagsString=__new0  BranchType=L  Resistance=1  Inductance=L  SetiL0=off  InitialCurrent=1  Capacitance=1e-6  Setx0=off  InitialVoltage=0  Measurements=None
  Series RLC Branch1 : powerlib/Elements/Series RLC Branch  LConnTagsString=__new0  RConnTagsString=__new0  BranchType=R  Resistance=5e3  Inductance=1e-3  SetiL0=off  InitialCurrent=0  Capacitance=15  Setx0=on  InitialVoltage=270  Measurements=None
  Unit Delay2 : UnitDelay  SampleTime=Ts  HasFrameUpgradeWarning=on
  Unit Delay3 : UnitDelay  SampleTime=Ts  HasFrameUpgradeWarning=on
  Voltage Measurement : powerlib/Measurements/Voltage Measurement  PhasorSimulation=off  OutputType=Complex  PSBequivalent=0
  Voltage Measurement1 : powerlib/Measurements/Voltage Measurement  PhasorSimulation=off  OutputType=Complex  PSBequivalent=0
  H+ : PMIOPort  Side=Right
  L+ : PMIOPort  Port=2  Side=Left
  H- : PMIOPort  Port=3  Side=Right
  L- : PMIOPort  Port=4  Side=Left
  IL : Outport
  VL : Outport  Port=2
  VH : Outport  Port=3
  IR : Outport  Port=4
  wires:
  D/1 -> [D]
  n/1 -> [n]
  [IL] -> IL/1
  [VL] -> VL/1
  [VH] -> VH/1
  [IR] -> IR/1
  [g] -> Ideal Switch1/1
  Fcn/1 -> Unit Delay2/1
  [D] -> Mux2/1
  Voltage Measurement/1 -> [VH]
  [VH] -> Mux1/2
  Current Measurement/1 -> [IL]
  [g] -> Ideal Switch3/1
  Unit Delay2/1 -> Cotrolled Voltage Source/1
  g/1 -> [g]
  Mux2/1 -> Fcn1/1
  Mux1/1 -> Fcn/1
  Current Measurement1/1 -> [IR]
  [IL] -> Mux2/2
  Fcn1/1 -> Unit Delay3/1
  [n] -> Mux2/3
  Unit Delay3/1 -> Controlled Current Source/1
  Voltage Measurement1/1 -> [VL]
  [D] -> Mux1/1
  connections:
  Diode2/RConn1 -- Series RLC Branch/LConn1
  Diode3/LConn1 -- Current Measurement1/RConn1
  Diode3/RConn1 -- Ideal Switch1/LConn1
  Series RLC Branch/RConn1 -- Current Measurement/LConn1
  Ideal Switch3/RConn1 -- Diode2/LConn1
  Current Measurement/RConn1 -- Cotrolled Voltage Source/RConn1
  Voltage Measurement/LConn2 -- H-/RConn1 -- L2/RConn1 -- L-/RConn1 -- Voltage Measurement1/LConn2 -- Cotrolled Voltage Source/LConn1 -- Controlled Current Source/LConn1 -- Series RLC Branch1/RConn1
  Controlled Current Source/RConn1 -- L2/LConn1 -- Current Measurement1/LConn1
  Voltage Measurement1/LConn1 -- Ideal Switch3/LConn1 -- L+/RConn1
  Voltage Measurement/LConn1 -- H+/RConn1 -- Ideal Switch1/RConn1 -- Series RLC Branch1/LConn1

== system lib_converters/Boost FC swh/Converter type/Swh ==
  g : Inport
  D : Inport  Port=2
  n : Inport  Port=3
  Current Measurement : powerlib/Measurements/Current Measurement  PhasorSimulation=off  OutputType=Complex  PSBequivalent=0
  Current Measurement1 : powerlib/Measurements/Current Measurement  PhasorSimulation=off  OutputType=Complex  PSBequivalent=0
  Diode1 : powerlib/Power Electronics/Diode  Ron=0.001  Lon=0  Vf=0  IC=0  UseSnubber=off  Rs=1e6  Cs=250e-9  Measurements=off
  Diode2 : powerlib/Power Electronics/Diode  Ron=0.001  Lon=0  Vf=0  IC=0  UseSnubber=off  Rs=1e6  Cs=250e-9  Measurements=off
  Diode3 : powerlib/Power Electronics/Diode  Ron=0.001  Lon=0  Vf=0  IC=0  UseSnubber=off  Rs=1e6  Cs=250e-9  Measurements=off
  Ideal Switch1 : powerlib/Power Electronics/Ideal Switch  Ron=0.001  Lon=0  IC=0  Rs=1e5  Cs=inf  Measurements=off
  Ideal Switch3 : powerlib/Power Electronics/Ideal Switch  Ron=0.001  Lon=0  IC=0  Rs=1e5  Cs=inf  Measurements=off
  L2 : powerlib/Elements/Series RLC Branch  LConnTagsString=__new0  RConnTagsString=__new0  BranchType=C  Resistance=0.01  Inductance=100e-6  SetiL0=off  InitialCurrent=100  Capacitance=Co  Setx0=off  InitialVoltage=100  Measurements=None
  Mosfet : powerlib/Power Electronics/Mosfet  Ron=0.1  Lon=0  Rd=0.01  Vfd=0  IC=0  Rs=1e5  Cs=inf  Measurements=on
  PWM Generator (DC-DC) : powerlib_meascontrol/Pulse & Signal Generators/PWM Generator (DC-DC)  Fsw=10000  Ts=Ts
  Series RLC Branch : powerlib/Elements/Series RLC Branch  LConnTagsString=__new0  RConnTagsString=__new0  BranchType=L  Resistance=1  Inductance=L  SetiL0=off  InitialCurrent=1  Capacitance=1e-6  Setx0=off  InitialVoltage=0  Measurements=None
  Series RLC Branch1 : powerlib/Elements/Series RLC Branch  LConnTagsString=__new0  RConnTagsString=__new0  BranchType=R  Resistance=5e3  Inductance=1e-3  SetiL0=off  InitialCurrent=0  Capacitance=15  Setx0=on  InitialVoltage=270  Measurements=None
  Voltage Measurement : powerlib/Measurements/Voltage Measurement  PhasorSimulation=off  OutputType=Complex  PSBequivalent=0
  Voltage Measurement1 : powerlib/Measurements/Voltage Measurement  PhasorSimulation=off  OutputType=Complex  PSBequivalent=0
  H+ : PMIOPort  Side=Right
  L+ : PMIOPort  Port=2  Side=Left
  H- : PMIOPort  Port=3  Side=Right
  L- : PMIOPort  Port=4  Side=Left
  IL : Outport
  VL : Outport  Port=2
  VH : Outport  Port=3
  IR : Outport  Port=4
  wires:
  PWM Generator (DC-DC)/1 -> Mosfet/1
  [D] -> PWM Generator (DC-DC)/1
  D/1 -> [D]
  Voltage Measurement1/1 -> [VL]
  n/1 -> [n]
  [g] -> Ideal Switch3/1
  Current Measurement/1 -> [IL]
  [IL] -> IL/1
  Voltage Measurement/1 -> [VH]
  g/1 -> [g]
  Current Measurement1/1 -> [IR]
  [g] -> Ideal Switch1/1
  [VL] -> VL/1
  [VH] -> VH/1
  [IR] -> IR/1
  connections:
  Diode3/LConn1 -- Current Measurement1/RConn1
  Diode3/RConn1 -- Ideal Switch1/LConn1
  Diode1/RConn1 -- L2/LConn1 -- Current Measurement1/LConn1
  Diode1/LConn1 -- Current Measurement/RConn1 -- Mosfet/LConn1
  Series RLC Branch/RConn1 -- Current Measurement/LConn1
  Ideal Switch3/RConn1 -- Diode2/LConn1
  Diode2/RConn1 -- Series RLC Branch/LConn1
  Series RLC Branch1/LConn1 -- Ideal Switch1/RConn1 -- H+/RConn1 -- Voltage Measurement/LConn1
  Ideal Switch3/LConn1 -- L+/RConn1 -- Voltage Measurement1/LConn1
  L2/RConn1 -- Mosfet/RConn1 -- L-/RConn1 -- Voltage Measurement1/LConn2 -- Series RLC Branch1/RConn1 -- H-/RConn1 -- Voltage Measurement/LConn2

== system lib_converters/Boost - PV/Control/Cascade-control/Discrete PI Controller3 ==
  note: Pierre Giroux, Gilbert Sybille
      | Power System Simulation Laboratory
      | IREQ, Hydro-Quebc
  note: Discrete PID Controller
  Error : Inport  SampleTime=Ts
  Discrete-Time Integrator : DiscreteIntegrator  InitialCondition=Init  SampleTime=Ts  LimitOutput=on  UpperSaturationLimit=UpperLimit  LowerSaturationLimit=LowerLimit  ICPrevOutput=DiscIntNeverNeededParam  ICPrevScaledInput=DiscIntNeverNeededParam
  Kp4 : Gain  Gain=Kp  SaturateOnIntegerOverflow=on  SampleTime=Ts  OutDataTypeStr=Inherit: Same as input  ParamDataTypeStr=Inherit: Same as input
  Kp5 : Gain  Gain=Ki  SaturateOnIntegerOverflow=on  SampleTime=Ts  OutDataTypeStr=Inherit: Same as input  ParamDataTypeStr=Inherit: Same as input
  Saturation2 : Saturate  UpperLimit=UpperLimit  LowerLimit=LowerLimit  SampleTime=Ts
  Sum6 : Sum  InputSameDT=on  SaturateOnIntegerOverflow=on  SampleTime=Ts  OutDataTypeStr=Inherit: Same as first input
  Zero-Order Hold : ZeroOrderHold  SampleTime=Ts
  Out : Outport  SampleTime=Ts  InitialOutput=0  VectorParamsAs1DForOutWhenUnconnected=off
  wires:
  Error/1 -> Kp4/1, Kp5/1
  Sum6/1 -> Saturation2/1
  Kp5/1 -> Discrete-Time Integrator/1
  Kp4/1 -> Zero-Order Hold/1
  Discrete-Time Integrator/1 -> Sum6/2
  Saturation2/1 -> Out/1
  Zero-Order Hold/1 -> Sum6/1

== system lib_converters/Boost - PV/Control/Cascade-control/Discrete PI Controller4 ==
  note: Discrete PID Controller
  note: Pierre Giroux, Gilbert Sybille
      | Power System Simulation Laboratory
      | IREQ, Hydro-Quebc
  Error : Inport  SampleTime=Ts
  Discrete-Time Integrator : DiscreteIntegrator  InitialCondition=Init  SampleTime=Ts  LimitOutput=on  UpperSaturationLimit=UpperLimit  LowerSaturationLimit=LowerLimit  ICPrevOutput=DiscIntNeverNeededParam  ICPrevScaledInput=DiscIntNeverNeededParam
  Kp4 : Gain  Gain=Kp  SaturateOnIntegerOverflow=on  SampleTime=Ts  OutDataTypeStr=Inherit: Same as input  ParamDataTypeStr=Inherit: Same as input
  Kp5 : Gain  Gain=Ki  SaturateOnIntegerOverflow=on  SampleTime=Ts  OutDataTypeStr=Inherit: Same as input  ParamDataTypeStr=Inherit: Same as input
  Saturation2 : Saturate  UpperLimit=UpperLimit  LowerLimit=LowerLimit  SampleTime=Ts
  Sum6 : Sum  InputSameDT=on  SaturateOnIntegerOverflow=on  SampleTime=Ts  OutDataTypeStr=Inherit: Same as first input
  Zero-Order Hold : ZeroOrderHold  SampleTime=Ts
  Out : Outport  SampleTime=Ts  InitialOutput=0  VectorParamsAs1DForOutWhenUnconnected=off
  wires:
  Zero-Order Hold/1 -> Sum6/1
  Saturation2/1 -> Out/1
  Discrete-Time Integrator/1 -> Sum6/2
  Kp4/1 -> Zero-Order Hold/1
  Kp5/1 -> Discrete-Time Integrator/1
  Sum6/1 -> Saturation2/1
  Error/1 -> Kp5/1, Kp4/1

== system lib_converters/Boost - PV - chsvar/Subsystem1/Subsystem1/Discrete PI Controller3 ==
  note: Pierre Giroux, Gilbert Sybille
      | Power System Simulation Laboratory
      | IREQ, Hydro-Quebc
  note: Discrete PID Controller
  Error : Inport  SampleTime=Ts
  Discrete-Time Integrator : DiscreteIntegrator  InitialCondition=Init  SampleTime=Ts  LimitOutput=on  UpperSaturationLimit=UpperLimit  LowerSaturationLimit=LowerLimit  ICPrevOutput=DiscIntNeverNeededParam  ICPrevScaledInput=DiscIntNeverNeededParam
  Kp4 : Gain  Gain=Kp  SaturateOnIntegerOverflow=on  SampleTime=Ts  OutDataTypeStr=Inherit: Same as input  ParamDataTypeStr=Inherit: Same as input
  Kp5 : Gain  Gain=Ki  SaturateOnIntegerOverflow=on  SampleTime=Ts  OutDataTypeStr=Inherit: Same as input  ParamDataTypeStr=Inherit: Same as input
  Saturation2 : Saturate  UpperLimit=UpperLimit  LowerLimit=LowerLimit  SampleTime=Ts
  Sum6 : Sum  InputSameDT=on  SaturateOnIntegerOverflow=on  SampleTime=Ts  OutDataTypeStr=Inherit: Same as first input
  Zero-Order Hold : ZeroOrderHold  SampleTime=Ts
  Out : Outport  SampleTime=Ts  InitialOutput=0  VectorParamsAs1DForOutWhenUnconnected=off
  wires:
  Error/1 -> Kp4/1, Kp5/1
  Sum6/1 -> Saturation2/1
  Kp5/1 -> Discrete-Time Integrator/1
  Kp4/1 -> Zero-Order Hold/1
  Discrete-Time Integrator/1 -> Sum6/2
  Saturation2/1 -> Out/1
  Zero-Order Hold/1 -> Sum6/1

== system lib_converters/Boost - PV - chsvar/Subsystem1/Subsystem1/Discrete PI Controller4 ==
  note: Discrete PID Controller
  note: Pierre Giroux, Gilbert Sybille
      | Power System Simulation Laboratory
      | IREQ, Hydro-Quebc
  Error : Inport  SampleTime=Ts
  Discrete-Time Integrator : DiscreteIntegrator  InitialCondition=Init  SampleTime=Ts  LimitOutput=on  UpperSaturationLimit=UpperLimit  LowerSaturationLimit=LowerLimit  ICPrevOutput=DiscIntNeverNeededParam  ICPrevScaledInput=DiscIntNeverNeededParam
  Kp4 : Gain  Gain=Kp  SaturateOnIntegerOverflow=on  SampleTime=Ts  OutDataTypeStr=Inherit: Same as input  ParamDataTypeStr=Inherit: Same as input
  Kp5 : Gain  Gain=Ki  SaturateOnIntegerOverflow=on  SampleTime=Ts  OutDataTypeStr=Inherit: Same as input  ParamDataTypeStr=Inherit: Same as input
  Saturation2 : Saturate  UpperLimit=UpperLimit  LowerLimit=LowerLimit  SampleTime=Ts
  Sum6 : Sum  InputSameDT=on  SaturateOnIntegerOverflow=on  SampleTime=Ts  OutDataTypeStr=Inherit: Same as first input
  Zero-Order Hold : ZeroOrderHold  SampleTime=Ts
  Out : Outport  SampleTime=Ts  InitialOutput=0  VectorParamsAs1DForOutWhenUnconnected=off
  wires:
  Zero-Order Hold/1 -> Sum6/1
  Saturation2/1 -> Out/1
  Discrete-Time Integrator/1 -> Sum6/2
  Kp4/1 -> Zero-Order Hold/1
  Kp5/1 -> Discrete-Time Integrator/1
  Sum6/1 -> Saturation2/1
  Error/1 -> Kp5/1, Kp4/1

== matlab function lib_converters/Bidirectional BOOST//BUCK - Batt/MATLAB Function5 ==
  settings: updateMethod=DISCRETE  sampleTime=Ts
  data: iL input; V output; VH input; D input; converter input; I output; n_boost input; n_buck input
function [V,I]= fcn(iL,VH,D,converter, n_boost, n_buck)
    
    if converter == 0
        V = VH*(1-D);
        I = iL*(1-D)*n_boost;
    else
        V = VH*D;
        I = iL*D/n_buck;
%         I = -iL*D/n_buck;
    end
    
end

== matlab function lib_converters/Boost - PV - chsvar/Subsystem1/MATLAB Function ==
  settings: updateMethod=DISCRETE  sampleTime=Ts
  data: u1 input; d output; mppt input; cascade input
function d = fcn(u1,mppt, cascade)
    if u1 == 1
        d = mppt;
    elseif u1 == 2
        d = cascade;
    else 
        d = mppt;
    end
end

== matlab function lib_converters/Boost - PV/Control/MPPT/MPPT ==
  settings: updateMethod=DISCRETE  sampleTime=Ts
  data: Vcom input; D output; Icom input; Vout input; Iout input; Vpv_in input; I_L input
function D  = PO(Vcom, Icom, Vout, Iout, Vpv_in, I_L)
    % MPPT controller based on the Perturb & Observe algorithm.
    
    % Dp:
    Dint = 0.5;
    Dmax = 0.9;
    Dmin = 0.1;
    deltaD = 1/5000;
    
    %% get previous value
    persistent Vpre Ppre Dpre Dirpre;
    dataType = 'double';
    
    %% init data
    if isempty(Dpre)
        Dpre = Dint;
        Vpre=0;
        Ppre=0;
        Dirpre=-1;
    end
    
    %% MPPT
    
%     Pout = Vout*Iout;
%     Pcom = Vcom*Icom;
    
    % Attention modif ici
    Pin = Vpv_in * I_L;
    Pout = Pin;
    
    Dir = 0;
    if Pout > Ppre
        Dir = 1;
    end
    if Pout < Ppre
        Dir = -1;
    end
    
    

    D = Dpre + Dir*deltaD;
    
    % If the power is lower than 0, it's not normal so we set the duty
    % cycle to its nominal value
    if Pout < 0
        if I_L >0
            D = Dint;
        end
    end

    
    %% Test if D above limits
    if D < Dmin
        D = Dmin;
    end
    if D > Dmax
        D = Dmax;
    end

    %% Save old data
    Dpre=D;
    Vpre=Vout;
    Ppre=Pout;
    Dirpre = Dir;

== matlab function lib_converters/Boost - PV - chsvar/Subsystem1/Subsystem/MPPT ==
  settings: updateMethod=DISCRETE  sampleTime=Ts
  data: Vcom input; D output; Icom input; Vout input; Iout input; Vpv_in input; I_L input
function D  = PO(Vcom, Icom, Vout, Iout, Vpv_in, I_L)
    % MPPT controller based on the Perturb & Observe algorithm.
    
    % Dp:
    Dint = 0.5;
    Dmax = 0.9;
    Dmin = 0.1;
    deltaD = 1/100000;
    
    %% get previous value
    persistent Vpre Ppre Dpre Dirpre;
    dataType = 'double';
    
    %% init data
    if isempty(Dpre)
        Dpre = Dint;
        Vpre=0;
        Ppre=0;
        Dirpre=-1;
    end
    
    %% MPPT
    
%     Pout = Vout*Iout;
%     Pcom = Vcom*Icom;
    
    % Attention modif ici
    Pin = Vpv_in * I_L;
    Pout = Pin;
    
    Dir = 0;
    if Pout > Ppre
        Dir = 1;
    end
    if Pout < Ppre
        Dir = -1;
    end
    
    

    D = Dpre + Dir*deltaD;
    
    % If the power is lower than 0, it's not normal so we set the duty
    % cycle to its nominal value
    if Pout < 0
        if I_L >0
            D = Dint;
        end
    end

    
    %% Test if D above limits
    if D < Dmin
        D = Dmin;
    end
    if D > Dmax
        D = Dmax;
    end

    %% Save old data
    Dpre=D;
    Vpre=Vout;
    Ppre=Pout;
    Dirpre = Dir;

== matlab function lib_converters/Bidirectional BOOST//BUCK - Batt - fast/MATLAB Function5 ==
  settings: updateMethod=DISCRETE  sampleTime=Ts
  data: iL input; V output; VH input; D input; converter input; I output; n_boost input; n_buck input
function [V,I]= fcn(iL,VH,D,converter, n_boost, n_buck)
    
    if converter == 0
        V = VH*(1-D);
        I = iL*(1-D)*n_boost;
    else
        V = VH*D;
        I = iL*D/n_buck;
%         I = -iL*D/n_buck;
    end
    
end

== matlab function lib_converters/Bidirectional BOOST//BUCK - avg-swh/Subsystem/avg/MATLAB Function5 ==
  settings: updateMethod=DISCRETE  sampleTime=Ts
  data: iL input; V output; VH input; D input; converter input; I output; n_boost input; n_buck input
function [V,I]= fcn(iL,VH,D,converter, n_boost, n_buck)
    
    if converter == 0
        V = VH*(1-D);
        I = iL*(1-D)*n_boost;
    else
        V = VH*D;
        I = iL*D/n_buck;
    end
    
end

== matlab function lib_converters/Boost - PV - fast/MPPT ==
  settings: updateMethod=DISCRETE  sampleTime=Ts
  data: D output; Vpv_in input; I_L input
function D  = PO(Vpv_in, I_L)
    % MPPT controller based on the Perturb & Observe algorithm.
    
    % Dp:
    Dint = 0.5;
    Dmax = 0.9;
    Dmin = 0.1;
    deltaD = 1/100000;
    
    %% get previous value
    persistent Ppre Dpre;
%     dataType = 'double';
    
    %% init data
    if isempty(Dpre)
        Dpre = Dint;
        Ppre=0;
    end
    
    %% MPPT
    
%     Pout = Vout*Iout;
%     Pcom = Vcom*Icom;
    
    % Attention modif ici
    Pin = Vpv_in * I_L;
    Pout = Pin;
    
    Dir = 0;
    if Pout > Ppre
        Dir = 1;
    end
    if Pout < Ppre
        Dir = -1;
    end
    
    

    D = Dpre + Dir*deltaD;
    
    % If the power is lower than 0, it's not normal so we set the duty
    % cycle to its nominal value
    if Pout < 0
        if I_L >0
            D = Dint;
        end
    end

    
    %% Test if D above limits
    if D < Dmin
        D = Dmin;
    end
    if D > Dmax
        D = Dmax;
    end

    %% Save old data
    Dpre=D;
    Ppre=Pout;
